simulink model "serial_connect"  (R2023a)
settings: Solver=VariableStepAuto  StartTime=0.0  StopTime=10.0  RelTol=1e-3
libraries: instrumentseriallib x2
settings Model: Creator=rhwns  LastModifiedBy=rhwns

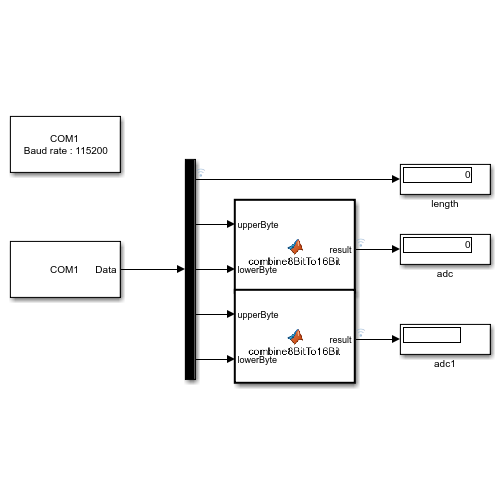
[thumbnail: Simulink's stored preview of the top-level diagram]
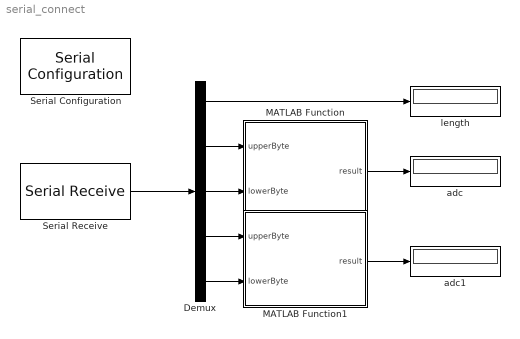
== system serial_connect ==
  Demux : Demux  Outputs=5
  MATLAB Function : MATLAB Function  TreatAsAtomicUnit=on
  MATLAB Function1 : MATLAB Function  TreatAsAtomicUnit=on
  Serial Configuration : instrumentseriallib/Serial Configuration  Priority=-200000  PortSel=COM1  Port=COM1  ComPort=COM1  BaudRate=115200  DataBits=8  Parity=none  StopBits=1  ByteOrder=little-endian  FlowControl=none  Timeout=10  SimulateUsing=Interpreted execution  BlockInModel=on  aMode=1
      settings: LibrarySourceBlock=embeddedtargetslib/Host Communication/Serial Configuration
  Serial Receive : instrumentseriallib/Serial Receive  Priority=1  PortSel=COM1  Port=COM1  ComPort=COM1  DataType=uint8  SaveDataType=uint8  ToggleHeader=on  Header=[0xFF 0xFF]  ToggleTerminator=on  Terminator=Custom terminator  CustomTerminator=[0x0A]  InputFormat=Column major  ToggleDataSize=on  DataSize=[5]  EnableBlockingMode=on  ActionDataUnavailable=Output last received value  ActionWhenDataUnavailable=Output last received value  CustomValue=0  SampleTime=0.01  SimulateUsing=Interpreted execution  BlockInModel=on  aMode=1
      settings: LibrarySourceBlock=embeddedtargetslib/Host Communication/Serial Receive
  adc : Display
  adc1 : Display
  length : Display
  wires:
  Serial Receive/1 -> Demux/1
  Demux/2 -> MATLAB Function/1(upperByte)
  Demux/3 -> MATLAB Function/2(lowerByte)
  Demux/1 -> length/1
  MATLAB Function/1(result) -> adc/1
  Demux/4 -> MATLAB Function1/1(upperByte)
  Demux/5 -> MATLAB Function1/2(lowerByte)
  MATLAB Function1/1(result) -> adc1/1

== matlab function serial_connect/MATLAB Function ==
  data: upperByte input; result output; lowerByte input
function result = combine8BitTo16Bit(upperByte, lowerByte)
    % 8비트 데이터를 16비트로 합칩니다.
    result = uint16(bitshift(uint16(upperByte), 8)) + uint16(lowerByte);
end

== matlab function serial_connect/MATLAB Function1 ==
  data: upperByte input; result output; lowerByte input
function result = combine8BitTo16Bit(upperByte, lowerByte)
    % 8비트 데이터를 16비트로 합칩니다.
    result = uint16(bitshift(uint16(upperByte), 8)) + uint16(lowerByte);
end
